simulink model "main"  (R2022a)
settings: Solver=ode4  StartTime=0.0  StopTime=20000  FixedStep=0.1  RelTol=1e-3
libraries: dspmathops x2
settings Model: Creator=sakur  LastModifiedBy=sakur

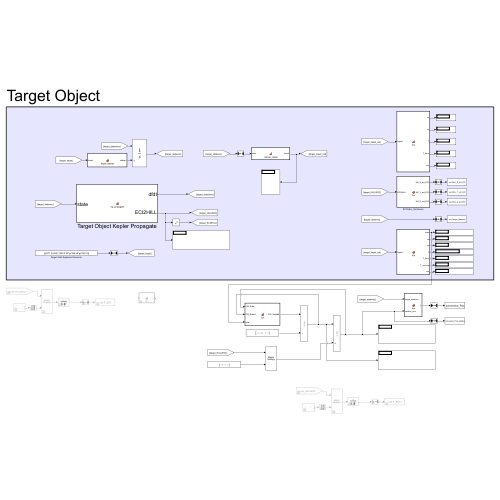
[thumbnail: Simulink's stored preview of the top-level diagram]
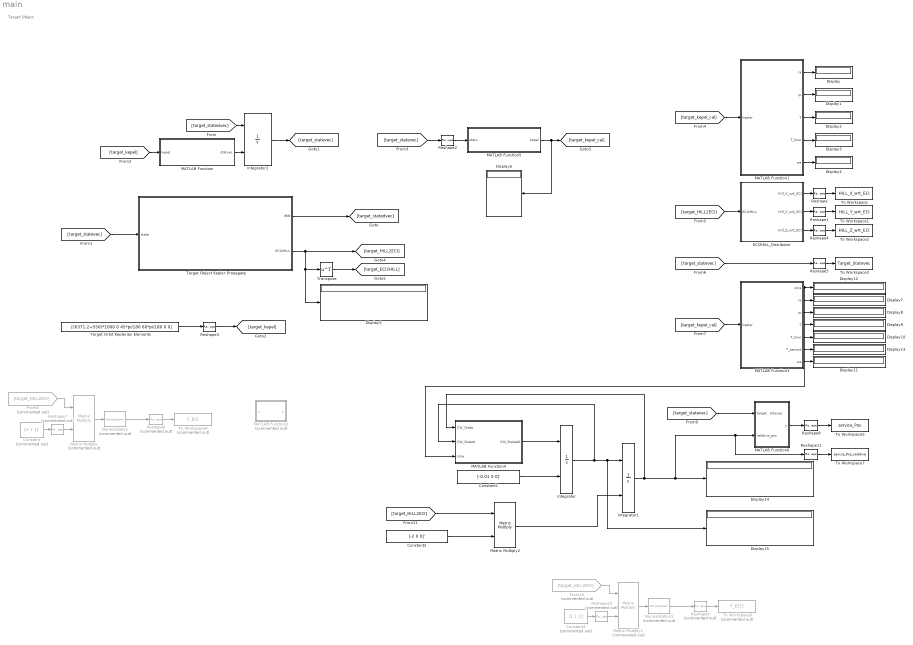
== system main ==
  note: Target Object
  Constant : Constant  Commented=on  Value=[1 1 1]'
  Constant1 : Constant  Value=[-0.01 0 0]'
  Constant2 : Constant  Value=[-2 0 0]'
  Constant3 : Constant  Commented=on  Value=[1 1 1]'
  Display{,1..15} (16 alike) : Display
  ECI2HILL_Distributor : MATLAB Function  TreatAsAtomicUnit=on
  From10 : From  Commented=on  GotoTag=target_HILL2ECI
  From8 : From  Commented=on  GotoTag=target_HILL2ECI
  Integrator : Integrator  InitialConditionSource=external
  Integrator1 : Integrator  InitialConditionSource=external
  Integrator2 : Integrator  InitialConditionSource=external  InitialCondition=[-7000 0 0 0 -9.175045 0 5233.5]'
  MATLAB Function : MATLAB Function  TreatAsAtomicUnit=on
  MATLAB Function1 : MATLAB Function  TreatAsAtomicUnit=on
  MATLAB Function2 : MATLAB Function  Commented=on  TreatAsAtomicUnit=on
  MATLAB Function3 : MATLAB Function  TreatAsAtomicUnit=on
  MATLAB Function4 : MATLAB Function  TreatAsAtomicUnit=on
  MATLAB Function5 : MATLAB Function  TreatAsAtomicUnit=on
  MATLAB Function6 : MATLAB Function  TreatAsAtomicUnit=on
  Matrix Multiply : Product  Commented=on  Multiplication=Matrix(*)
  Matrix Multiply1 : Product  Commented=on  Multiplication=Matrix(*)
  Matrix Multiply2 : Product  Multiplication=Matrix(*)
  Normalization : dspmathops/Normalization  Commented=on  NormType=Squared 2-norm  Bias=1e-10  NormOver=Each column  Dimension=1  roundingMode=Floor  overflowMode=off  accumDataTypeStr=Inherit: Same as product output  accumLastDataTypeStr=Inherit: Same as product output  outputDataTypeStr=Inherit: Same as product output  outputMin=[]  outputMax=[]  outputLastDataTypeStr=Inherit: Same as product output
  Normalization1 : dspmathops/Normalization  Commented=on  NormType=Squared 2-norm  Bias=1e-10  NormOver=Each column  Dimension=1  roundingMode=Floor  overflowMode=off  accumDataTypeStr=Inherit: Same as product output  accumLastDataTypeStr=Inherit: Same as product output  outputDataTypeStr=Inherit: Same as product output  outputMin=[]  outputMax=[]  outputLastDataTypeStr=Inherit: Same as product output
  Reshape{,1..5,8,11} (8 alike) : Reshape  OutputDimensionality=Row vector (2-D)
  Reshape10 : Reshape  Commented=on  OutputDimensionality=Column vector (2-D)
  Reshape6 : Reshape  Commented=on  OutputDimensionality=Row vector (2-D)
  Reshape7 : Reshape  Commented=on  OutputDimensionality=Column vector (2-D)
  Reshape9 : Reshape  Commented=on  OutputDimensionality=Row vector (2-D)
  Target Object Kepler Propagate : MATLAB Function  TreatAsAtomicUnit=on
  Target Orbit Keplerian Elements : Constant  Value=[(6371.2+550)*1000 0 45*pi/180 60*pi/180 0 0]
  To Workspace : ToWorkspace  VariableName=HILL_X_wrt_ECI  SampleTime=-1
      settings: Save2DSignal=2-D array (concatenate along first dimension)
  To Workspace1 : ToWorkspace  VariableName=HILL_Y_wrt_ECI  SampleTime=-1
      settings: Save2DSignal=2-D array (concatenate along first dimension)
  To Workspace2 : ToWorkspace  VariableName=HILL_Z_wrt_ECI  SampleTime=-1
      settings: Save2DSignal=2-D array (concatenate along first dimension)
  To Workspace3 : ToWorkspace  VariableName=Target_Statevec  SampleTime=-1
      settings: Save2DSignal=2-D array (concatenate along first dimension)
  To Workspace4 : ToWorkspace  Commented=on  VariableName=F_ECI  SampleTime=-1
      settings: Save2DSignal=2-D array (concatenate along first dimension)
  To Workspace5 : ToWorkspace  VariableName=service_Pos  SampleTime=-1
      settings: Save2DSignal=2-D array (concatenate along first dimension)
  To Workspace6 : ToWorkspace  Commented=on  VariableName=F_ECI1  SampleTime=-1
      settings: Save2DSignal=2-D array (concatenate along first dimension)
  To Workspace7 : ToWorkspace  VariableName=sevice_Pos_relative  SampleTime=-1
      settings: Save2DSignal=2-D array (concatenate along first dimension)
  Transpose : Math  Operator=transpose
  wires:
  Reshape2/1 -> MATLAB Function5/1(statv)
  MATLAB Function/1(statvec) -> Integrator2/2
  Target Object Kepler Propagate/1(dfdt) -> [target_statedvec]
  [target_statedvec] -> Integrator2/1
  Integrator2/1 -> [target_statevec]
  [target_statevec] -> Target Object Kepler Propagate/1(state)
  Reshape3/1 -> [target_kepel]
  Target Orbit Keplerian Elements/1 -> Reshape3/1
  [target_kepel] -> MATLAB Function/1(kepel)
  [target_statevec] -> Reshape2/1
  MATLAB Function5/1(kepel) -> Display6/1, [target_kepel_cal]
  [target_kepel_cal] -> MATLAB Function1/1(kepler)
  MATLAB Function1/1(ra) -> Display/1
  MATLAB Function1/2(rp) -> Display1/1
  MATLAB Function1/4(T_hour) -> Display3/1
  MATLAB Function1/3(T) -> Display2/1
  MATLAB Function1/5(we) -> Display4/1
  Target Object Kepler Propagate/2(ECI2HILL) -> Transpose/1, Display5/1, [target_HILL2ECI]
  [target_HILL2ECI] -> ECI2HILL_Distributor/1(ECI2HILL)
  ECI2HILL_Distributor/1(Hill_X_wrt_ECI) -> Reshape/1
  Reshape/1 -> To Workspace/1
  Reshape1/1 -> To Workspace1/1
  Reshape4/1 -> To Workspace2/1
  ECI2HILL_Distributor/3(Hill_Z_wrt_ECI) -> Reshape4/1
  ECI2HILL_Distributor/2(Hill_Y_wrt_ECI) -> Reshape1/1
  Reshape5/1 -> To Workspace3/1
  [target_statevec] -> Reshape5/1
  MATLAB Function3/2(ra) -> Display7/1
  MATLAB Function3/3(rp) -> Display8/1
  MATLAB Function3/5(T_hour) -> Display10/1
  MATLAB Function3/4(T) -> Display9/1
  MATLAB Function3/7(we) -> Display11/1
  [target_kepel_cal] -> MATLAB Function3/1(kepler)
  MATLAB Function3/1(sma) -> MATLAB Function4/3(sma), Display12/1
  MATLAB Function3/6(T_second) -> Display13/1
  Transpose/1 -> [target_ECI2HILL]
  Reshape6/1 -> To Workspace4/1
  Matrix Multiply/1 -> Normalization/1
  Constant/1 -> Reshape7/1
  From8/1 -> Matrix Multiply/1
  Reshape7/1 -> Matrix Multiply/2
  Normalization/1 -> Reshape6/1
  MATLAB Function4/1(CW_Statedd) -> Integrator/1
  Integrator1/1 -> Reshape11/1, MATLAB Function6/2(relative_pos), Display14/1, MATLAB Function4/1(CW_State)
  Constant1/1 -> Integrator/2
  [target_statevec] -> MATLAB Function6/1(target_statevec)
  MATLAB Function6/1(y) -> Reshape8/1
  Reshape8/1 -> To Workspace5/1
  Normalization1/1 -> Reshape9/1
  From10/1 -> Matrix Multiply1/1
  Reshape9/1 -> To Workspace6/1
  Matrix Multiply1/1 -> Normalization1/1
  Constant3/1 -> Reshape10/1
  Reshape10/1 -> Matrix Multiply1/2
  [target_HILL2ECI] -> Matrix Multiply2/1
  Constant2/1 -> Matrix Multiply2/2
  Matrix Multiply2/1 -> Integrator1/2
  Integrator/1 -> MATLAB Function4/2(CW_Stated), Display15/1, Integrator1/1
  Reshape11/1 -> To Workspace7/1

== matlab function main/MATLAB Function2 ==
  data: u input; y output
function y = fcn(u)

y = u;

== matlab function main/MATLAB Function1 ==
  data: kepler input; ra output; rp output; T output; T_hour output; we output
function [ra, rp, T, T_hour, we] = fcn(kepler)

u=3.9865*10^14;

a = kepler(1);
e = kepler(2);
% 

ra = a*(1+e);%장반경
rp = a*(1-e);%단반경

a = (ra+rp)/2;% semi-major axis

% a = (550 + 6371.8)*1000;

T = 2*pi*sqrt((a*a*a)/(u));

T_hour = T/3600;

we = 2*pi/T;
% we = 1.1207*0.001;

end

== matlab function main/ECI2HILL_Distributor ==
  data: Hill_X_wrt_ECI output; ECI2HILL input; Hill_Y_wrt_ECI output; Hill_Z_wrt_ECI output
function [Hill_X_wrt_ECI, Hill_Y_wrt_ECI, Hill_Z_wrt_ECI] = fcn(ECI2HILL)

Hill_X_wrt_ECI = ECI2HILL(:,1);
Hill_Y_wrt_ECI = ECI2HILL(:,2);
Hill_Z_wrt_ECI = ECI2HILL(:,3);


end

== matlab function main/Target Object Kepler Propagate ==
  data: state input; dfdt output; ECI2HILL output
function [dfdt, ECI2HILL]  = eq_propagate(state)
% Lectures_TwoBodyProblem.pdf
% 우주시스템입문 - 도미타 노부유키 eq(7.8) p136
% https://en.wikipedia.org/wiki/Standard_gravitational_parameter
u  = 3.9865*10^14; % earth gravitional parameter
Re = 6378137;      % earth radius [m]

dfdt = zeros(size(state));

% x=x
% x1=dx/dt
% dx1/dt = d^2(x)/dt

x  = state(1); % x
y  = state(2); % y
z  = state(3); % z
x1 = state(4); % x1 = dx/dt
y1 = state(5); % y1 = dy/dt
z1 = state(6); % z1 = dz/dt

r = [x,y,z]';
v = [x1,y1,z1]';

r_norm=sqrt(x^2+y^2+z^2);

% % %   Keplar Motion Equatnion
% % %  => r_dd + u/(r^3)r_ = 0 => r_dd = -u/(r^3)r_
dfdt(1) = x1;
dfdt(2) = y1;
dfdt(3) = z1;
dfdt(4) = -u*x/r_norm^3;
dfdt(5) = -u*y/r_norm^3;
dfdt(6) = -u*z/r_norm^3;

% % % get Hill Frame
h = cross(r, v);
Hill_X = r/norm(r);
Hill_Z = h/norm(h);
Hill_Y = cross(Hill_Z, Hill_X);

ECI2HILL = [Hill_X, Hill_Y, Hill_Z];

end

== matlab function main/MATLAB Function3 ==
  data: sma output; kepler input; ra output; rp output; T output; T_hour output; T_second output; we output
function [sma, ra, rp, T, T_hour, T_second, we] = fcn(kepler)

u=3.9865*10^14;

sma = kepler(1);
a   = kepler(1);
e   = kepler(2);
% 

ra = a*(1+e);%장반경
rp = a*(1-e);%단반경

a = (ra+rp)/2;% semi-major axis

% a = (550 + 6371.8)*1000;

T = 2*pi*sqrt((a*a*a)/(u));

T_hour   = T/3600;
T_second = T;
we       = 2*pi/T;
% we = 1.1207*0.001;

end

== matlab function main/MATLAB Function ==
  data: kepel input; statvec output
function statvec  = kepel_statvec (kepel)
%  [statvec] = kepel_statvec (kepel)
%	The function kepel_statvec transforms the keplerian
%	elements kepel into the corresponding state vector in
%	the same reference system.
%
% Input:
%	kepel
% 		vector containing the keplerian elements:
%		(1) - semimajor axis of the orbit in meters.
%		(2) - eccentricity.
%		(3) - inclinatsion in radians.
%		(4) - right ascension of ascending node in radians.
%		(5) - argument of perigee in radians.
%		(6) - mean anomaly in radians.
% Output:
%	statvec
%  		state vector in meters and meters/second.
%
% Authors:
%	Helio K. Kuga;
%	Valder M. Medeiros;
%	Valdemir Carrara		february/80		version 1.0
%	Valdemir Carrara		july 2005		(C version)
%   Valdemir Carrara            March/09        Matlab

EARTH_GRAVITY	= 3.9860064e+14;		% Earth's gravitational constant (m**3/s**2)

a    = kepel(1);	% semi-major axis
exc  = kepel(2);	% eccentricity

c1   = sqrt(1. - exc*exc);

%     rotation matrix

orb2iner = rotmaz(-kepel(4))*rotmax(-kepel(3))*rotmaz(-kepel(5));

%     Kepler's equation

E    = kepler(kepel(6), exc);

sE   = sin(E);
cE   = cos(E);
c3   = sqrt(EARTH_GRAVITY/a)/(1. - exc*cE);

%     state vector

statvec = [[a*(cE - exc), a*c1*sE, 0]*orb2iner', [-c3*sE, c1*c3*cE, 0]*orb2iner'];

end

function [rot_mat] = rotmax (angle)
% [rot_mat] = rotmax (angle)
%   To obtain the rotation matrix around the X axis given the
%   rotation angle.
% inputs:
%   angle
%       rotation angle, in radians.
% outputs:
%   rot_mat
%       rotation matrix (3, 3)
%

% Valdemir Carrara, Sep, 1998

coan    =  cos(angle);
sian    =  sin(angle);

rot_mat =  [1, 0, 0; 0, coan, sian; 0, -sian, coan];

end

function [rot_mat] = rotmay (angle)
% [rot_mat] = rotmay (angle)
%   To obtain the rotation matrix around the Y axis given the
%   rotation angle.
% inputs:
%   angle
%       rotation angle, in radians.
% outputs:
%   rot_mat
%       rotation matrix (3, 3)
%

% Valdemir Carrara, Sep, 1998


coan    =  cos(angle);
sian    =  sin(angle);

rot_mat =  [coan, 0, -sian; 0, 1, 0; sian, 0, coan];

end

function [rot_mat] = rotmaz (angle)
% [rot_mat] = rotmaz (angle)
%   To obtain the rotation matrix around the Z axis given the
%   rotation angle.
% inputs:
%   angle
%       rotation angle, in radians.
% outputs:
%   rot_mat
%       rotation matrix (3, 3)
%

% Valdemir Carrara, Sep, 1998

coan    =  cos(angle);
sian    =  sin(angle);

rot_mat =  [coan, sian, 0; -sian, coan, 0; 0, 0, 1];
end

function [eccentric] = kepler (mean_anomaly, eccentricity)
% [eccentric] = kepler (mean_anomaly, eccentricity)
%	The subroutine kepler finds a solution to the
%	kepler's equation.
%
% Input:
%	mean_anomaly
%		mean anomaly in radians.
%	eccentricity
%		eccentricity.
%
% Output:
%	eccentric
%		eccentric anomaly in radians.
%
% Authors:
%	Valder M. de Medeiros		june/81		version 2.0
%	Valdemir Carrara			july 2005	(C version)
%   Valdemir Carrara            March/09        Matlab

exc2    = eccentricity*eccentricity;
am1     = mod (mean_anomaly, 2*pi);
am2     = am1 + am1;
am3     = am1 + am2;
shoot   = am1 + eccentricity*(1. - 0.125*exc2)*sin(am1) + ...
		0.5*exc2*(sin(am2) + 0.75*eccentricity*sin(am3));
shoot   = mod (shoot, 2*pi);

e1      = 1.0;
ic      = 0;

while ((abs(e1) > 1.e-12) && (ic <= 10)) 
	e1    = (shoot - am1 - eccentricity*sin(shoot)) / ...
			(1.0 - eccentricity*cos(shoot));
    shoot = shoot - e1;
    ic    = ic + 1;
end

if (ic >= 10)
    disp ('warning ** subroutine kepler did not converge in 10 iterations');
end

eccentric = shoot;


end

== matlab function main/MATLAB Function4 ==
  data: CW_State input; CW_Statedd output; CW_Stated input; sma input
function CW_Statedd = fcn(CW_State, CW_Stated, sma)

x  = CW_State(1);
y  = CW_State(2);
z  = CW_State(3);
xd = CW_Stated(1);
yd = CW_Stated(2);
zd = CW_Stated(3);

mu = 3.986005*10^14;
n = sqrt(mu/(sma*sma*sma));

F = [100 100 100]';
a = F./1;
% % Clohessy-Wiltshire Equation
xdd =  3*n*n*x + 2*n*yd + a(1);
ydd = -2*n*xd + a(2);
zdd = -n*n*z + a(3);

CW_Statedd = [xdd, ydd, zdd]';

end

== matlab function main/MATLAB Function6 ==
  data: target_statevec input; relative_pos input; y output
function y = fcn(target_statevec, relative_pos)
y = [target_statevec(1), target_statevec(2), target_statevec(3)]' + ...
    [relative_pos(1), relative_pos(2), relative_pos(3)]';
end

== matlab function main/MATLAB Function5 ==
  settings: updateMethod=DISCRETE
  data: statv input; kepel output
function kepel  = statvec_kepel (statv)
%	The function statvec_kepel transforms the state vector statv
%	into the corresponding keplerian elements in the
%	same reference system.
%
% Input:
%	statv
%		state vector in meters and meters/second.
%
% Output:
%	statvec_kepel
%		vector containing the keplerian elements:
%		(1) - semimajor axis of the orbit in meters.
%		(2) - eccentricity.
%		(3) - inclination in radians.
%		(4) - right ascension of ascending node in radians.
%		(5) - argument of perigee in radians.
%		(6) - mean anomaly in radians.

EARTH_GRAVITY	= 3.9860064e+14;		% Earth's gravitational constant (m**3/s**2)

    xp     = [statv(1),statv(2),statv(3)];
    xv     = [statv(4),statv(5),statv(6)];
    r      = sqrt(xp*xp');
    vq     = xv*xv';
    ainv   = 2.0/(r) - vq/EARTH_GRAVITY;

    h      = cross(xp, xv);
    hm     = sqrt(h*h');
    if (hm < 1.e-10)
        disp (' *** Message from function statvec_kepel: *** ');
        disp (' There are no keplerian elements corresponding to this state vector');
        kepel = [0, 0, 0, 0, 0, 0];
    else
        h      = h/hm;
        incl   = acos(h(3));
        raan   = atan2(h(1), -h(2));
        d      = xp*xv' / EARTH_GRAVITY;
        esene  = d * sqrt(EARTH_GRAVITY*ainv);
        ecose  = 1 - r*ainv;
        exc    = sqrt(esene*esene + ecose*ecose);
        E      = atan2(esene, ecose);
        mean   = mod (E - esene, 2*pi);
        an = [0 0 0];
        if mean < 0
            mean = mean + 2*pi;
        end
        if exc < 1.e-10
            arpe = 0;
        else
            dp     = 1./r - ainv;
            ev     = dp*xp - d*xv;
            abev   = sqrt(ev*ev');
            ev     = ev/abev;
            an(1)  = cos(raan);
            an(2)  = sin(raan);
            an(3)  = 0;
            fi     = ev*cross(h, an)';
            arpe = acos(ev*an');
            if fi < 0
                arpe  =  -arpe + 2*pi;
            end
        end

        kepel = [(1./ainv), exc, incl, raan, arpe, mean];
    end



end
